simulink model "FOC_w_LTID_v2"  (R2018b)
settings: Solver=ode5  StartTime=0  StopTime=16  FixedStep=1/fs/4  MaxStep=1/fs  RelTol=1e-5  EnableMultiTasking=on
InitFcn:
  | controllers
  | model_parameters
  | KT2C = 1/(3/2)/(Npp*Lndmpm);
  | Tload = 10;
  | noise_ena = 1;
  | 
  | %SMO
  | SMO_load_gain = 15*1;  %15 corresponds to 1040
  | SMO_gain_p = 2; %1 corresponds to 70
  | smo_load_phi = 50;
  | smo_load_esf = 25; %25
  | smo_load_cutoff = 55; %75 %Hz
values from neighbouring files (symbols this model uses):
  B_m = 0.0016655    [model_parameters.m]
  C_m = 0.2295    [model_parameters.m]
  fs = 1*5e3    (= 5000)    [model_parameters.m]
  gamma = 0.001    [model_parameters.m]
  i_maxim_PM = 35    [model_parameters.m]
  J = 0.0146    [model_parameters.m]
  Ld = 2.2e-3    (= 0.0022)    [model_parameters.m]
  Lndd_ini = Lndmpm    (= 0.12258)    [model_parameters.m]
  Lndmpm = 0.12258    [model_parameters.m]
  Lq = 2.2e-3    (= 0.0022)    [model_parameters.m]
  Npp = 4    [model_parameters.m]
  Omegae_ini = 0    [model_parameters.m]
  Rs = 0.268*1    (= 0.268)    [model_parameters.m]
  Tl_const = Trat/nrat^2    (= 6.91358024691e-07)    [model_parameters.m]
  Vph = Vs*sqrt(2)    [model_parameters.m]
undefined symbols (not defined in the file or in its folder): DiscIntNeverNeededParam, Ka_speed, Ki_id, Ki_iq, Ki_speed, Kp_id, Kp_iq, Kp_speed, sigbuilder_block
libraries: simulink x2
settings Model: Creator=klu  LastModifiedBy=Barna
settings DataIOCC: LimitDataPoints=on  SaveFormat=Array  SignalLoggingSaveFormat=ModelDataLogs
settings OptimizationCC: BooleanDataType=off  ExpressionDepthLimit=2147483647  InitFltsAndDblsToZero=on  LifeSpan=inf
settings DebuggingCC: AlgebraicLoopMsg=none  SaveWithParameterizedLinksMsg=none  UnderspecifiedInitializationDetection=Classic  MergeDetectMultiDrivingBlocksExec=none  SignalResolutionControl=TryResolveAllWithWarning  MultiTaskDSMMsg=warning  MultiTaskCondExecSysMsg=none  FcnCallInpInsideContextMsg=warning  StateNameClashWarn=warning  SFUnexpectedBacktrackingDiag=warning  SFNoUnconditionalDefaultTransitionDiag=warning  SFExecutionAtInitializationDiag=none
settings HardwareCC: ProdBitPerPointer=32  ProdBitPerSizeT=32  ProdBitPerPtrDiffT=32  ProdLargestAtomicFloat=None  ProdIntDivRoundTo=Undefined  ProdEndianess=Unspecified  ProdWordSize=32  ProdHWDeviceType=32-bit Generic
settings ModelReferenceCC: PropagateSignalLabelsOutOfModel=off
settings SFSimCC: SimUseLocalCustomCode=off
settings RTWCC: RTWUseLocalCustomCode=off
settings CodeAppCC: StateflowObjectComments=on
settings GRTTargetCC: TargetFcnLib=ansi_tfl_tmw.mat  TargetLangStandard=C89/C90 (ANSI)  GeneratePreprocessorConditionals=Disable all  CombineOutputUpdateFcns=off  GRTInterface=on
settings ConfigComp: CovMetricSettings=dw  CovHtmlReporting=on  CovSaveCumulativeToWorkspaceVar=on  CovSaveSingleToWorkspaceVar=on  CovExternalEMLEnable=off  CovSFcnEnable=off

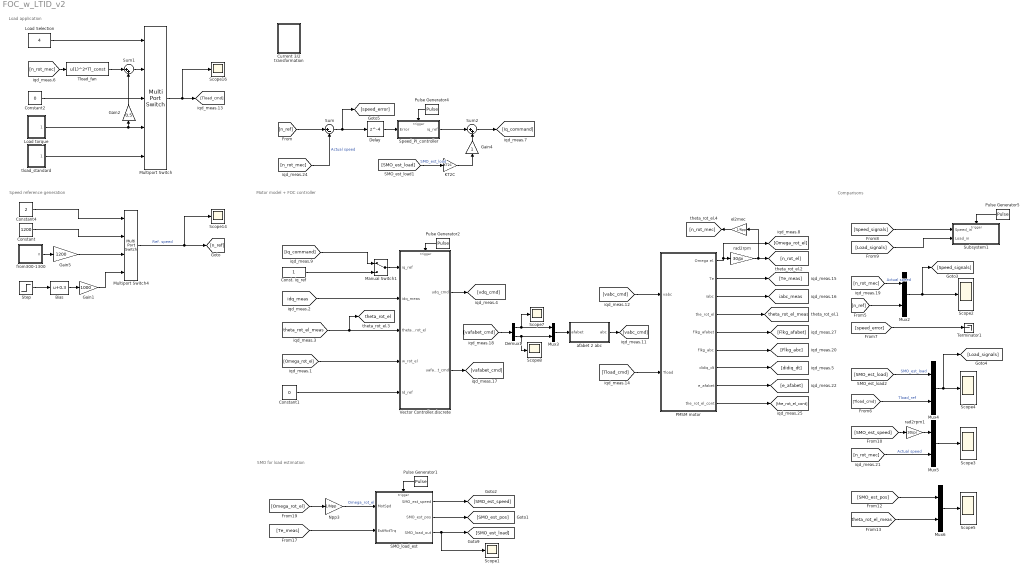
== system FOC_w_LTID_v2 ==
  note: Speed reference generation
  note: Motor model + FOC controller
  note: Load application
  note: SMO for load estimation
  note: Comparisons
  Bias : Bias  Bias=0.3
  Const. iq_ref : Constant
  Constant : Constant  Value=1200
  Constant1 : Constant  Value=0
  Constant2 : Constant  Value=0
  Constant4 : Constant  Value=2
  Current 3/2 transformation : Subsystem
      mask Display:
      | plot([0.1000    0.1357    0.1714    0.2071    0.2429    0.2786    0.3143    0.3500    0.3857    0.4214 0.4571    0.4929    0.5286    0.5643    0.6000]-0.05,0.4+0.6*[0.5000    0.5868    0.6564    0.6950    0.6950    0.6564    0.5868    0.5000    0.4132    0.3436 0.3050    0.3050    0.3436    0.4132    0.5000])
      | 
      | plot([0.1,0.9],[0.1,0.9])
      | 
      | plot([0.5,0.9],0.3*[1 1])
  Delay : Delay  DelayLength=4
  Demux1 : Demux  Outputs=2
  Gain1 : Gain  Gain=1000
  Gain2 : Gain  Gain=0.5
  Gain4 : Gain
  Gain5 : Gain  Gain=1200
  KT2C : Gain  Gain=KT2C
  Load Selection : Constant  Value=4
  Load torque : Subsystem
  Manual Switch1 : ManualSwitch
  Multiport Switch : MultiPortSwitch  Inputs=4
  Multiport Switch4 : MultiPortSwitch
  Mux{2..6} (5 alike) : Mux  Inputs=2
  Npp3 : Gain  Gain=1/Npp
  PMSM motor : Subsystem
  Pulse Generator1 : DiscretePulseGenerator  PulseType=Time based  Period=1/fs  PulseWidth=50
  Pulse Generator2 : DiscretePulseGenerator  PulseType=Time based  Period=1/fs  PulseWidth=50
  Pulse Generator4 : DiscretePulseGenerator  PulseType=Time based  Period=1/fs*2  PulseWidth=50
  Pulse Generator5 : DiscretePulseGenerator  PulseType=Time based  Period=1/fs  PulseWidth=50
  SMO_load_est : Subsystem
  Scope{1..5,7..8,14,16} (9 alike) : Scope
  Speed_PI_controller : Subsystem
  Step : Step  SampleTime=0
  Subsystem1 : Subsystem
  Sum : Sum  Inputs=|+-
  Sum1 : Sum  Inputs=|++
  Sum2 : Sum  Inputs=|++
  Terminator1 : Terminator
  Tload_fan : Fcn  Expr=u(1)^2*Tl_const
  Vector Controller.discrete : Subsystem
  afabet 2 abc : Subsystem
  el2mec : Gain  Gain=1/Npp
  "from300-1300 " : Subsystem  Tag=STV Subsys  LoadFcn=sigbuilder_block('load');  StartFcn=sigbuilder_block('start');  StopFcn=sigbuilder_block('stop');  ClipboardFcn=sigbuilder_block('clipboard');  mask(Sigbuilder block){tuvar=[0:10]}
      mask help: Sigbuilder GUI
      mask init:
      | if ~strcmp(get_param(bdroot(gcbh),'SimulationStatus'),'stopped') tuvar = sigbuilder_block('maskInit'); end
      settings: CopyFcn=sigbuilder_block('copy');  DeleteFcn=sigbuilder_block('delete');  ModelCloseFcn=sigbuilder_block('modelClose');  PreSaveFcn=sigbuilder_block('preSave');  PauseFcn=sigbuilder_block('pause')  ContinueFcn=sigbuilder_block('continue')  NameChangeFcn=sigbuilder_block('namechange');  OpenFcn=sigbuilder_block('open',[0 0 1096.2 591.6 ]);  CloseFcn=sigbuilder_block('close');
      mask Display: plot(0, 0, 100, 100,[2, 2, 32, 32, 2], [68, 8, 8, 68, 68],[32, 2], [38, 38], [32, 19, 2],[53, 60, 44], [32, 17, 17, 2],[16, 16, 31, 31]);txt = getActiveGroup(gcbh);text(2, 100, txt,'verticalAlignment', 'top');
  rad2rpm : Gain  Gain=30/pi
  rad2rpm1 : Gain  Gain=30/pi
  tload_standard : Subsystem
  tag scope: iabc_meas=global, theta_rot_el=global, theta_rot_el_meas=global
  wires:
  Manual Switch1/1 -> Vector Controller.discrete/1(iq_ref)
  Const. iq_ref/1 -> Manual Switch1/2
  [idq_meas] -> Vector Controller.discrete/2(idq_meas)
  Vector Controller.discrete/1(udq_cmd) -> [vdq_cmd]
  Vector Controller.discrete/2(uafabet_cmd) -> [vafabet_cmd]
  Constant2/1 -> Multiport Switch/3
  Load torque/1(T_load) -> Multiport Switch/4, Gain2/1
  Multiport Switch/1 -> Scope16/1, [Tload_cmd]
  [n_rot_mec] -> Tload_fan/1
  Load Selection/1 -> Multiport Switch/1
  Pulse Generator2/1 -> Vector Controller.discrete/Trigger
  Sum1/1 -> Multiport Switch/2
  Tload_fan/1 -> Sum1/1
  Constant1/1 -> Vector Controller.discrete/5(Id_ref)
  Gain2/1 -> Sum1/2
  PMSM motor/2(Te) -> [Te_meas]
  PMSM motor/1(Omega el.) -> [Omega_rot_el], rad2rpm/1
  [vabc_cmd] -> PMSM motor/1(vabc)
  rad2rpm/1 -> el2mec/1, [n_rot_el]
  PMSM motor/4(the_rot_el) -> [theta_rot_el_meas]
  PMSM motor/5(Flkg_afabet) -> [Flkg_afabet]
  PMSM motor/6(Flkg_abc) -> [Flkg_abc]
  [Tload_cmd] -> PMSM motor/2(Tload)
  PMSM motor/3(iabc) -> [iabc_meas]
  PMSM motor/7(didiq_dt) -> [didiq_dt]
  Demux1/2 -> Mux3/2, Scope8/1
  Demux1/1 -> Scope7/1, Mux3/1
  [vafabet_cmd] -> Demux1/1
  afabet 2 abc/1(abc) -> [vabc_cmd]
  Mux3/1 -> afabet 2 abc/1(afabet)
  el2mec/1 -> [n_rot_mec]
  [Iq_command] -> Manual Switch1/1
  [theta_rot_el_meas] -> [theta_rot_el], Vector Controller.discrete/3(theta_rot_el)
  [Omega_rot_el] -> Vector Controller.discrete/4(w_rot_el)
  PMSM motor/8(e_afabet) -> [e_afabet]
  Multiport Switch4/1 -> Scope14/1, [n_ref]  "Ref. speed"
  Pulse Generator4/1 -> Speed_PI_controller/Trigger
  Sum/1 -> Delay/1, [speed_error]
  Constant4/1 -> Multiport Switch4/1
  Constant/1 -> Multiport Switch4/2
  PMSM motor/9(the_rot_el_cont) -> [the_rot_el_cont]
  Delay/1 -> Speed_PI_controller/1(Error)
  tload_standard/1(T_load) -> Multiport Switch/5
  "from300-1300 "/1(n) -> Gain5/1
  [n_rot_mec] -> Sum/2  "Actual speed"
  [n_ref] -> Sum/1
  Gain5/1 -> Multiport Switch4/3
  Step/1 -> Bias/1
  Bias/1 -> Gain1/1
  Gain1/1 -> Multiport Switch4/4
  [Omega_rot_el] -> Npp3/1
  [Te_meas] -> SMO_load_est/2(EstMotTrq)
  Npp3/1 -> SMO_load_est/1(MotSpd)  "Omega_rot_el"
  Pulse Generator1/1 -> SMO_load_est/Trigger
  Speed_PI_controller/1(iq_ref) -> Sum2/1
  Sum2/1 -> [Iq_command]
  Gain4/1 -> Sum2/2
  [SMO_est_load] -> KT2C/1  "SMO_est_load"
  KT2C/1 -> Gain4/1
  [speed_error] -> Terminator1/1
  Mux4/1 -> Scope4/1, [Load_signals]
  [SMO_est_load] -> Mux4/1  "SMO_est_load"
  [Tload_cmd] -> Mux4/2  "Tload_ref"
  Mux2/1 -> [Speed_signals], Scope2/1
  [Speed_signals] -> Subsystem1/1(Speed_in)
  [Load_signals] -> Subsystem1/2(Load_in)
  Pulse Generator5/1 -> Subsystem1/Trigger
  [theta_rot_el_meas] -> Mux6/2
  [n_ref] -> Mux2/2
  [SMO_est_pos] -> Mux6/1
  [n_rot_mec] -> Mux2/1  "Actual speed"
  Mux5/1 -> Scope3/1
  [n_rot_mec] -> Mux5/2  "Actual speed"
  [SMO_est_speed] -> rad2rpm1/1
  rad2rpm1/1 -> Mux5/1
  Mux6/1 -> Scope5/1
  SMO_load_est/2(SMO_est_pos) -> [SMO_est_pos]
  SMO_load_est/1(SMO_est_speed) -> [SMO_est_speed]
  SMO_load_est/3(SMO_load_out) -> Scope1/1, [SMO_est_load]

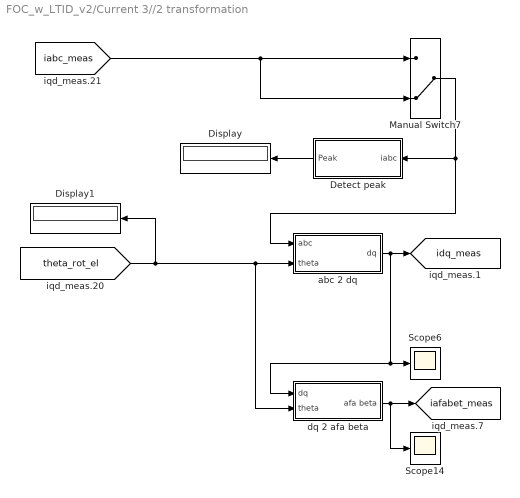
== system FOC_w_LTID_v2/Current 3//2 transformation ==
  Detect peak : Subsystem
  Display : Display
  Display1 : Display
  Manual Switch7 : ManualSwitch  CurrentSetting=0
  Scope14 : Scope
  Scope6 : Scope
  abc 2 dq : Subsystem
  dq 2 afa beta : Subsystem
  tag scope: iafabet_meas=global, idq_meas=global
  wires:
  abc 2 dq/1(dq) -> [idq_meas], Scope6/1, dq 2 afa beta/1(dq)
  dq 2 afa beta/1(afa beta) -> [iafabet_meas], Scope14/1
  Manual Switch7/1 -> abc 2 dq/1(abc), Detect peak/1(iabc)
  Detect peak/1(Peak) -> Display/1
  [theta_rot_el] -> abc 2 dq/2(theta), dq 2 afa beta/2(theta), Display1/1
  [iabc_meas] -> Manual Switch7/1, Manual Switch7/2

== system FOC_w_LTID_v2/Load torque ==
  Add : Sum  Inputs=+++
  Step Load torque 1 : Step  Time=1.5  After=Tload  SampleTime=0
  Step Load torque2 : Step  Time=2  After=-Tload  SampleTime=0
  Tload : Constant  Value=0
  T_load : Outport
  wires:
  Tload/1 -> Add/1
  Step Load torque 1/1 -> Add/2
  Step Load torque2/1 -> Add/3
  Add/1 -> T_load/1

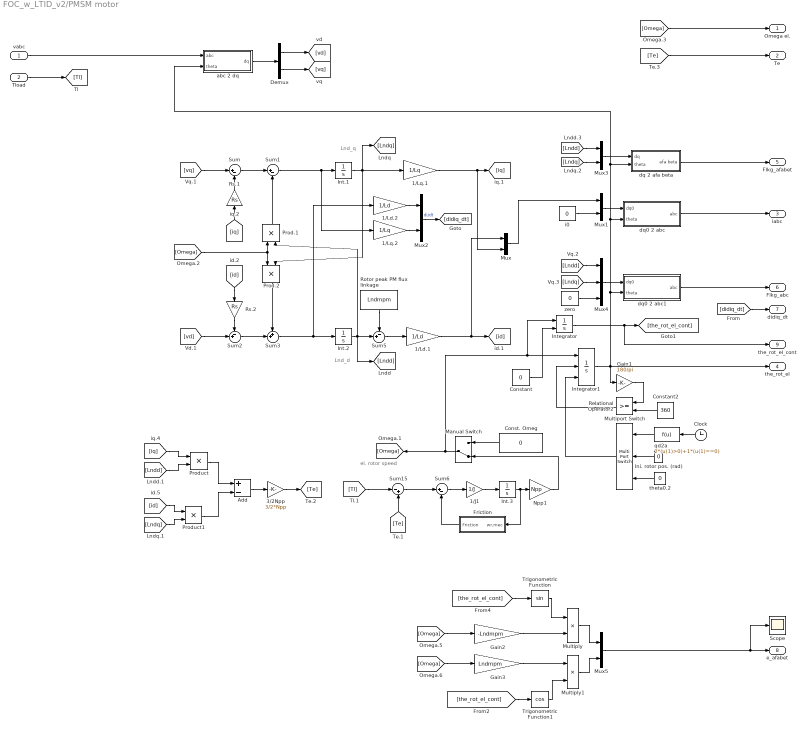
== system FOC_w_LTID_v2/PMSM motor ==
  note: Lnd_d
  note: Lnd_q
  note: el. rotor speed
  vabc : Inport
  Tload : Inport  Port=2
  1/J1 : Gain  Gain=1/J
  1/Ld.1 : Gain  Gain=1/Ld
  1/Ld.2 : Gain  Gain=1/Ld
  1/Lq.1 : Gain  Gain=1/Lq
  1/Lq.2 : Gain  Gain=1/Lq
  3/2Npp : Gain  Gain=3/2*Npp
  Add : Sum  Inputs=+-
  Clock : Clock
  Const. Omeg : Constant  Value=0
  Constant : Constant  Value=0
  Constant2 : Constant  Value=360
  Demux : Demux  Outputs=2
  Friction : Subsystem
  Gain1 : Gain  Gain=180/pi
  Gain2 : Gain  Gain=-Lndmpm
  Gain3 : Gain  Gain=Lndmpm
  Ini. rotor pos. (rad) : Constant  Value=0
  Int.1 : Integrator
  Int.2 : Integrator  InitialCondition=Lndd_ini
  Int.3 : Integrator  InitialCondition=Omegae_ini/Npp
  Integrator : Integrator  InitialConditionSource=external
  Integrator1 : Integrator  ExternalReset=rising  InitialConditionSource=external  InitialCondition=pi/3
  Manual Switch : ManualSwitch  CurrentSetting=0
  Multiply : Product
  Multiply1 : Product
  Multiport Switch : MultiPortSwitch  Inputs=2
  Mux{,1..3,5} (5 alike) : Mux  Inputs=2
  Mux4 : Mux  Inputs=3
  Npp1 : Gain  Gain=Npp
  Prod.1 : Product  RndMeth=Zero
  Prod.2 : Product  RndMeth=Zero
  Product : Product  RndMeth=Zero
  Product1 : Product  RndMeth=Zero
  Relational Operator2 : RelationalOperator  OutDataTypeStr=boolean  RndMeth=Nearest
  Rotor peak PM flux linkage : Constant  Value=Lndmpm
  Rs.1 : Gain  Gain=Rs
  Rs.2 : Gain  Gain=Rs
  Scope : Scope
  Sum : Sum  Inputs=|+-
  Sum1 : Sum  Inputs=|+-
  Sum15 : Sum  Inputs=|-+
  Sum2 : Sum  Inputs=-+|
  Sum3 : Sum  Inputs=++|
  Sum5 : Sum  Inputs=-+|
  Sum6 : Sum  Inputs=|+-
  Trigonometric Function : Trigonometry
  Trigonometric Function1 : Trigonometry  Operator=cos
  abc 2 dq : Subsystem
  dq 2 afa beta : Subsystem
  dq0 2 abc : Subsystem
  dq0 2 abc1 : Subsystem
  i0 : Constant  Value=0
  qd2a : Fcn  Expr=2*(u(1)>0)+1*(u(1)==0)
  theta0.2 : Constant  Value=0
  zero : Constant  Value=0
  Omega el. : Outport
  Te : Outport  Port=2
  iabc : Outport  Port=3
  the_rot_el : Outport  Port=4
  Flkg_afabet : Outport  Port=5
  Flkg_abc : Outport  Port=6
  didiq_dt : Outport  Port=7
  e_afabet : Outport  Port=8
  the_rot_el_cont : Outport  Port=9
  wires:
  3/2Npp/1 -> [Te]
  Add/1 -> 3/2Npp/1
  Sum5/1 -> 1/Ld.1/1
  Rotor peak PM flux linkage/1 -> Sum5/1
  [Omega] -> Omega el./1
  [Te] -> Te/1
  Product1/1 -> Add/2
  Product/1 -> Add/1
  [Lndq] -> Product1/2
  [id] -> Product1/1
  [Te] -> Sum15/2
  [Tl] -> Sum15/1
  Mux/1 -> Mux1/1
  [Omega] -> Prod.2/1, Prod.1/1
  Sum3/1 -> Int.2/1, 1/Ld.2/1
  Prod.2/1 -> Sum3/1
  Sum2/1 -> Sum3/2
  [id] -> Rs.2/1
  Rs.2/1 -> Sum2/1
  [vd] -> Sum2/2
  1/Ld.1/1 -> [id], Mux/1
  Int.2/1 -> [Lndd], Sum5/2, Prod.1/2
  [iq] -> Rs.1/1
  1/Lq.1/1 -> [iq], Mux/2
  Prod.1/1 -> Sum1/2
  Sum1/1 -> Int.1/1, 1/Lq.2/1
  Int.1/1 -> 1/Lq.1/1, Prod.2/2, [Lndq]
  Sum/1 -> Sum1/1
  Rs.1/1 -> Sum/2
  [vq] -> Sum/1
  Tload/1 -> [Tl]
  Demux/2 -> [vq]
  Demux/1 -> [vd]
  i0/1 -> Mux1/2
  Mux1/1 -> dq0 2 abc/1(dq0)
  dq0 2 abc/1(abc) -> iabc/1
  vabc/1 -> abc 2 dq/1(abc)
  abc 2 dq/1(dq) -> Demux/1
  Integrator1/1 -> the_rot_el/1, dq0 2 abc/2(theta), dq 2 afa beta/2(theta), abc 2 dq/2(theta), dq0 2 abc1/2(theta), Gain1/1
  1/Ld.2/1 -> Mux2/1
  1/Lq.2/1 -> Mux2/2
  Mux3/1 -> dq 2 afa beta/1(dq)
  [Lndd] -> Mux3/1
  [Lndq] -> Mux3/2
  dq 2 afa beta/1(afa beta) -> Flkg_afabet/1
  [Lndd] -> Mux4/1
  [Lndq] -> Mux4/2
  Mux4/1 -> dq0 2 abc1/1(dq0)
  dq0 2 abc1/1(abc) -> Flkg_abc/1
  zero/1 -> Mux4/3
  Gain1/1 -> Relational Operator2/1
  Constant2/1 -> Relational Operator2/2
  [iq] -> Product/1
  [Lndd] -> Product/2
  Relational Operator2/1 -> Integrator1/2
  Ini. rotor pos. (rad)/1 -> Multiport Switch/2
  theta0.2/1 -> Multiport Switch/3
  qd2a/1 -> Multiport Switch/1
  Clock/1 -> qd2a/1
  Multiport Switch/1 -> Integrator1/3
  Const. Omeg/1 -> Manual Switch/1
  Npp1/1 -> Manual Switch/2
  Manual Switch/1 -> Integrator/1, Integrator1/1, [Omega]
  Friction/1(Friction) -> Sum6/2
  Int.3/1 -> Friction/1(wr,mec), Npp1/1
  Sum6/1 -> 1/J1/1
  1/J1/1 -> Int.3/1
  Sum15/1 -> Sum6/1
  Mux5/1 -> Scope/1, e_afabet/1
  Trigonometric Function1/1 -> Multiply1/2
  [Omega] -> Gain2/1
  [the_rot_el_cont] -> Trigonometric Function1/1
  Gain3/1 -> Multiply1/1
  Multiply1/1 -> Mux5/2
  [the_rot_el_cont] -> Trigonometric Function/1
  Multiply/1 -> Mux5/1
  [Omega] -> Gain3/1
  Gain2/1 -> Multiply/2
  Trigonometric Function/1 -> Multiply/1
  Integrator/1 -> the_rot_el_cont/1, [the_rot_el_cont]
  Constant/1 -> Integrator/2
  Mux2/1 -> [didiq_dt]  "di/dt"
  [didiq_dt] -> didiq_dt/1

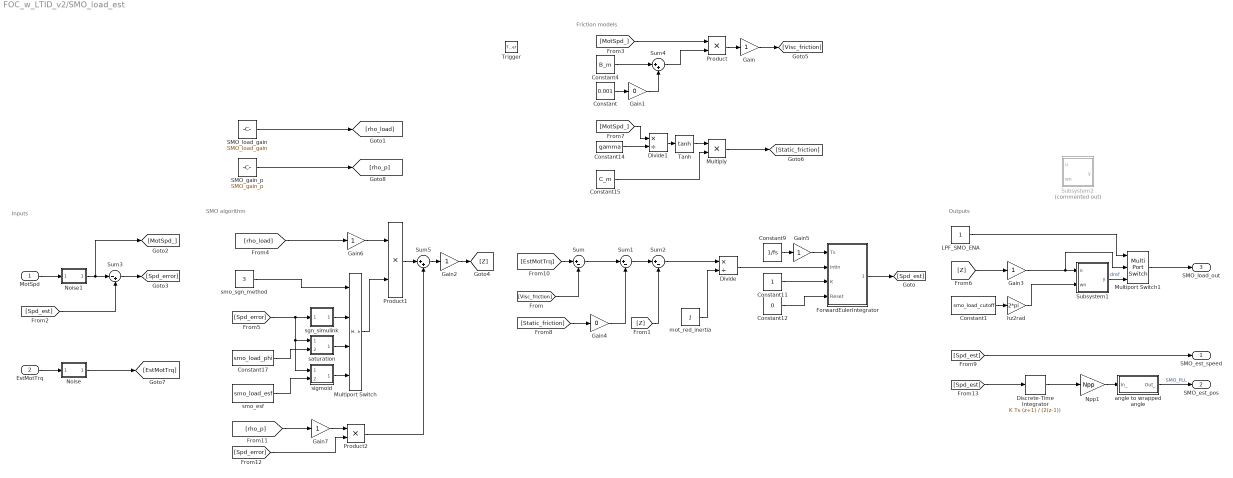
== system FOC_w_LTID_v2/SMO_load_est ==
  note: Inputs
  note: Outputs
  note: Friction models
  note: SMO algorithm
  MotSpd : Inport
  EstMotTrq : Inport  Port=2
  Trigger : TriggerPort  VariantControl=(inherit)
  Constant : Constant  Value=0.001
  Constant1 : Constant  Value=smo_load_cutoff
  Constant11 : Constant
  Constant12 : Constant  Value=0
  Constant14 : Constant  Value=gamma
  Constant15 : Constant  Value=C_m
  Constant17 : Constant  Value=smo_load_phi
  Constant4 : Constant  Value=B_m
  Constant9 : Constant  Value=1/fs
  Discrete-Time Integrator : DiscreteIntegrator  IntegratorMethod=Integration: Trapezoidal  SampleTime=-1  ICPrevOutput=DiscIntNeverNeededParam  ICPrevScaledInput=DiscIntNeverNeededParam
  Divide : Product  Inputs=*/
  Divide1 : Product  Inputs=*/
  ForwardEulerIntegrator : Subsystem
  Gain{,2..3,5..7} (6 alike) : Gain
  Gain1 : Gain  Gain=0
  Gain4 : Gain  Gain=0
  LPF_SMO_ENA : Constant
  Multiply : Product
  Multiport Switch : MultiPortSwitch
  Multiport Switch1 : MultiPortSwitch  DataPortOrder=Zero-based contiguous  Inputs=2  zeroidx=on
  Noise : Subsystem
  Noise1 : Subsystem
  Npp1 : Gain  Gain=Npp
  Product : Product
  Product1 : Product
  Product2 : Product
  SMO_gain_p : Constant  Value=SMO_gain_p
  SMO_load_gain : Constant  Value=SMO_load_gain
  Subsystem1 : Subsystem
  Subsystem2 : Subsystem  Commented=on
  Sum : Sum  Inputs=|+-
  Sum1 : Sum  Inputs=|+-
  Sum2 : Sum  Inputs=|+-
  Sum3 : Sum  Inputs=|-+
  Sum4 : Sum  Inputs=|++
  Sum5 : Sum  Inputs=|++
  Tanh : Trigonometry  Operator=tanh
  angle to wrapped angle : Subsystem
  hz2rad : Gain  Gain=2*pi
  mot_red_inertia : Constant  Value=J
  saturation : Subsystem
  sgn_simulink : Subsystem
  sigmoid : Subsystem
  smo_esf : Constant  Value=smo_load_esf
  smo_sgn_method : Constant  Value=3
  SMO_est_speed : Outport
  SMO_est_pos : Outport  Port=2
  SMO_load_out : Outport  Port=3
  wires:
  [Visc_friction] -> Sum/2
  Sum/1 -> Sum1/1
  mot_red_inertia/1 -> Divide/2
  [Spd_est] -> Sum3/2
  MotSpd/1 -> Noise1/1(In1)
  Sum3/1 -> [Spd_error]
  Product/1 -> Gain/1
  [MotSpd_] -> Product/1
  Gain/1 -> [Visc_friction]
  Constant4/1 -> Sum4/1
  Constant/1 -> Gain1/1
  Gain1/1 -> Sum4/2
  Sum4/1 -> Product/2
  Gain2/1 -> [Z]
  [rho_load] -> Gain6/1
  smo_sgn_method/1 -> Multiport Switch/1
  sgn_simulink/1(Out_) -> Multiport Switch/2
  saturation/1(Out_) -> Multiport Switch/3
  sigmoid/1(Out_) -> Multiport Switch/4
  Multiport Switch/1 -> Product1/2
  Constant17/1 -> saturation/2(phi)
  smo_esf/1 -> sigmoid/2(esf)
  [Spd_error] -> sgn_simulink/1(Sigma), sigmoid/1(Sigma), saturation/1(Sigma)
  Constant1/1 -> hz2rad/1
  Gain3/1 -> Multiport Switch1/2, Subsystem1/1(u)
  hz2rad/1 -> Subsystem1/2(wn)
  Constant14/1 -> Divide1/2
  Constant15/1 -> Multiply/2
  Divide1/1 -> Tanh/1
  Tanh/1 -> Multiply/1
  [MotSpd_] -> Divide1/1
  Multiply/1 -> [Static_friction]
  [Static_friction] -> Gain4/1
  Gain4/1 -> Sum1/2
  Constant12/1 -> ForwardEulerIntegrator/4(Reset)
  Constant11/1 -> ForwardEulerIntegrator/3(K)
  Constant9/1 -> Gain5/1
  Gain5/1 -> ForwardEulerIntegrator/1(Ts)
  ForwardEulerIntegrator/1(IntOut_) -> [Spd_est]
  Subsystem1/1(y) -> Multiport Switch1/3  "dref"
  Multiport Switch1/1 -> SMO_load_out/1
  LPF_SMO_ENA/1 -> Multiport Switch1/1
  [Spd_est] -> SMO_est_speed/1
  EstMotTrq/1 -> Noise/1(In1)
  [EstMotTrq] -> Sum/1
  SMO_load_gain/1 -> [rho_load]
  Noise/1(Out1) -> [EstMotTrq]
  Noise1/1(Out1) -> [MotSpd_], Sum3/1
  Sum1/1 -> Sum2/1
  Sum2/1 -> Divide/1
  Divide/1 -> ForwardEulerIntegrator/2(IntIn)
  [Z] -> Sum2/2
  [Z] -> Gain3/1
  Product1/1 -> Sum5/1
  Sum5/1 -> Gain2/1
  [rho_p] -> Gain7/1
  [Spd_error] -> Product2/2
  Product2/1 -> Sum5/2
  SMO_gain_p/1 -> [rho_p]
  Npp1/1 -> angle to wrapped angle/1(In_)
  Discrete-Time Integrator/1 -> Npp1/1
  [Spd_est] -> Discrete-Time Integrator/1
  angle to wrapped angle/1(Out_) -> SMO_est_pos/1  "SMO_PLL"
  Gain6/1 -> Product1/1
  Gain7/1 -> Product2/1

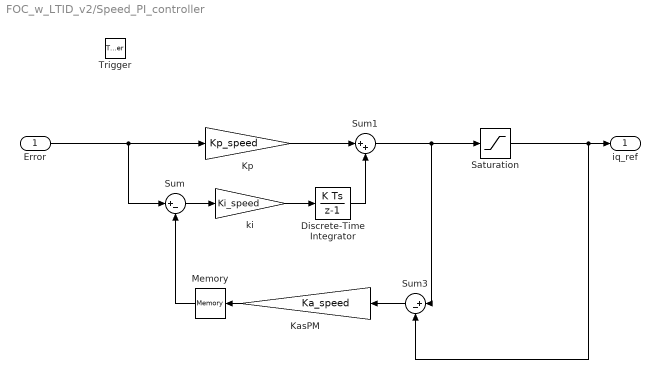
== system FOC_w_LTID_v2/Speed_PI_controller ==
  Error : Inport
  Trigger : TriggerPort  VariantControl=(inherit)
  Discrete-Time Integrator : DiscreteIntegrator  SampleTime=-1  ICPrevOutput=DiscIntNeverNeededParam  ICPrevScaledInput=DiscIntNeverNeededParam
  KasPM : Gain  Gain=Ka_speed
  Kp : Gain  Gain=Kp_speed
  Memory : Memory  InheritSampleTime=on
  Saturation : Saturate  UpperLimit=i_maxim_PM  LowerLimit=-i_maxim_PM
  Sum : Sum  Inputs=|+-
  Sum1 : Sum  Inputs=|++
  Sum3 : Sum  Inputs=|+-
  ki : Gain  Gain=Ki_speed
  iq_ref : Outport
  wires:
  Kp/1 -> Sum1/1
  ki/1 -> Discrete-Time Integrator/1
  Discrete-Time Integrator/1 -> Sum1/2
  Error/1 -> Sum/1, Kp/1
  KasPM/1 -> Memory/1
  Memory/1 -> Sum/2
  Sum1/1 -> Sum3/1, Saturation/1
  Sum3/1 -> KasPM/1
  Saturation/1 -> iq_ref/1, Sum3/2
  Sum/1 -> ki/1

== system FOC_w_LTID_v2/Subsystem1 ==
  Speed_in : Inport
  Load_in : Inport  Port=2
  Trigger : TriggerPort  VariantControl=Variant  PortDimensions=1
  To Workspace : ToWorkspace  VariableName=Speed_in  SaveFormat=Structure With Time  SampleTime=-1
  To Workspace1 : ToWorkspace  VariableName=SMO_EstLoad  SaveFormat=Structure With Time  SampleTime=-1
  wires:
  Speed_in/1 -> To Workspace/1
  Load_in/1 -> To Workspace1/1

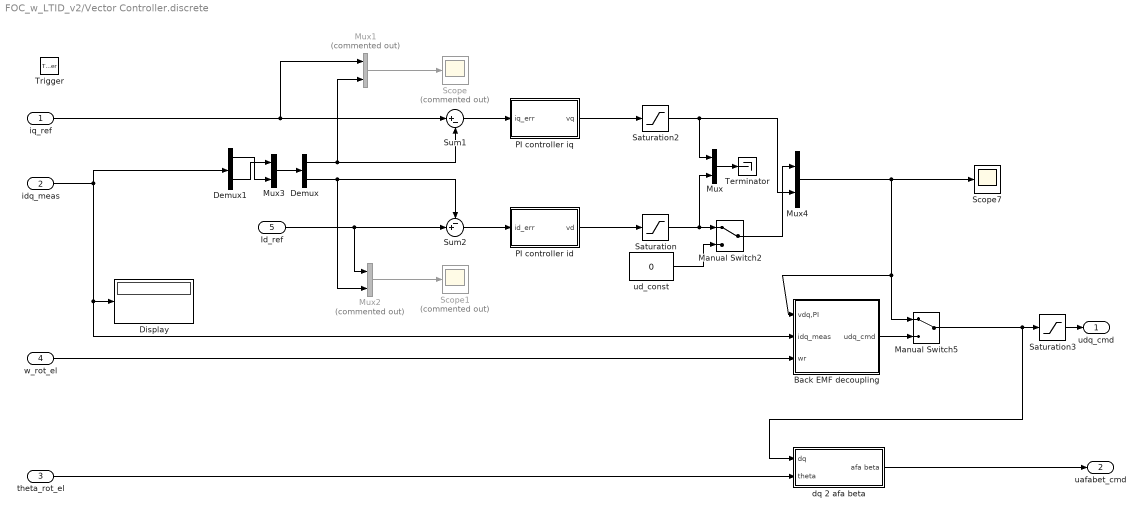
== system FOC_w_LTID_v2/Vector Controller.discrete ==
  iq_ref : Inport
  idq_meas : Inport  Port=2
  theta_rot_el : Inport  Port=3
  w_rot_el : Inport  Port=4
  Id_ref : Inport  Port=5
  Trigger : TriggerPort  VariantControl=(inherit)
  Back EMF decoupling : Subsystem
  Demux : Demux  Outputs=2
  Demux1 : Demux  Outputs=2
  Display : Display
  Manual Switch2 : ManualSwitch
  Manual Switch5 : ManualSwitch
  Mux : Mux  Inputs=2
  Mux1 : Mux  Commented=on  Inputs=2
  Mux2 : Mux  Commented=on  Inputs=2
  Mux3 : Mux  Inputs=2
  Mux4 : Mux  Inputs=2
  PI controller id : Subsystem
  PI controller iq : Subsystem
  Saturation : Saturate  UpperLimit=Vph  LowerLimit=-Vph
  Saturation2 : Saturate  UpperLimit=Vph  LowerLimit=-Vph
  Saturation3 : Saturate  UpperLimit=Vph  LowerLimit=-Vph
  Scope : Scope  Commented=on
  Scope1 : Scope  Commented=on
  Scope7 : Scope
  Sum1 : Sum  Inputs=|+-
  Sum2 : Sum  Inputs=-+|
  Terminator : Terminator
  dq 2 afa beta : Subsystem
  ud_const : Constant  Value=0
  udq_cmd : Outport
  uafabet_cmd : Outport  Port=2
  wires:
  Id_ref/1 -> Sum2/2, Mux2/1
  Saturation/1 -> Mux/2, Manual Switch2/1
  Mux/1 -> Terminator/1
  PI controller iq/1(vq) -> Saturation2/1
  Demux/1 -> Sum1/2, Mux1/2
  PI controller id/1(vd) -> Saturation/1
  Demux/2 -> Sum2/1, Mux2/2
  Sum1/1 -> PI controller iq/1(iq_err)
  Sum2/1 -> PI controller id/1(id_err)
  iq_ref/1 -> Sum1/1, Mux1/1
  Saturation2/1 -> Mux/1, Mux4/2
  Manual Switch2/1 -> Mux4/1
  ud_const/1 -> Manual Switch2/2
  Demux1/2 -> Mux3/1
  Demux1/1 -> Mux3/2
  theta_rot_el/1 -> dq 2 afa beta/2(theta)
  w_rot_el/1 -> Back EMF decoupling/3(wr)
  Back EMF decoupling/1(udq_cmd) -> Manual Switch5/2
  Mux4/1 -> Scope7/1, Manual Switch5/1, Back EMF decoupling/1(vdq,PI)
  Manual Switch5/1 -> dq 2 afa beta/1(dq), Saturation3/1
  Mux3/1 -> Demux/1
  idq_meas/1 -> Demux1/1, Display/1, Back EMF decoupling/2(idq_meas)
  Saturation3/1 -> udq_cmd/1
  dq 2 afa beta/1(afa beta) -> uafabet_cmd/1
  Mux1/1 -> Scope/1
  Mux2/1 -> Scope1/1

== system FOC_w_LTID_v2/afabet 2 abc ==
  afabet : Inport
  Constant : Constant  Value=0
  Mux1 : Mux  Inputs=2
  Mux2 : Mux  Inputs=3
  qd2a : Fcn  Expr=u(1)+u(3)
  qd2b : Fcn  Expr=u(1)*cos(2/3*pi)+u(2)*sin(2/3*pi)+u(3)
  qd2c : Fcn  Expr=u(1)*cos(2/3*pi)-u(2)*sin(2/3*pi)+u(3)
  abc : Outport
  wires:
  Constant/1 -> Mux1/2
  qd2c/1 -> Mux2/3
  afabet/1 -> Mux1/1
  Mux1/1 -> qd2c/1, qd2b/1, qd2a/1
  qd2a/1 -> Mux2/1
  qd2b/1 -> Mux2/2
  Mux2/1 -> abc/1

== system FOC_w_LTID_v2/from300-1300  ==
  Demux : Demux  Tag=STV Demux  Outputs=1
  FromWs : FromWorkspace  Tag=STV FromWs  VariableName=tuvar  SampleTime=0
      SigBuilderData=|
      | common.afterFinalStr = 'Extrapolate'
      | common.sampleTime = 0
      | dataSet.timeRange = [0 16]
      | dataSet.name = 'Group 1'
      | sbobj.Groups.Name = 'Group 1'
      | sbobj.Groups.Signals.Name = 'n'
      | sbobj.Groups.Signals.XData = [0 1 1.5 5 5.5 11 11.5 15 15.5 16]
      | sbobj.Groups.Signals.YData = [0.3 0.3 1.3 1.3 0.3 0.3 1.3 1.3 0.3 0.3]
      | sbobj.Groups.TimeRange = [0 16]
  n : Outport  Tag=STV Outport
  wires:
  Demux/1 -> n/1
  FromWs/1 -> Demux/1

== system FOC_w_LTID_v2/tload_standard ==
  Add : Sum  Inputs=+++++
  Step Load torque 1 : Step  Time=3  After=Tload  SampleTime=0
  Step Load torque1 : Step  Time=9  After=Tload  SampleTime=0
  Step Load torque2 : Step  Time=7  After=-Tload  SampleTime=0
  Step Load torque3 : Step  Time=13  After=-Tload  SampleTime=0
  Tload_ini : Constant  Value=0
  T_load : Outport
  wires:
  Tload_ini/1 -> Add/1
  Step Load torque 1/1 -> Add/2
  Step Load torque2/1 -> Add/3
  Add/1 -> T_load/1
  Step Load torque1/1 -> Add/4
  Step Load torque3/1 -> Add/5

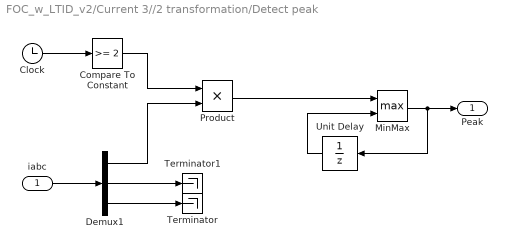
== system FOC_w_LTID_v2/Current 3//2 transformation/Detect peak ==
  iabc : Inport
  Clock : Clock
  Compare To Constant : simulink/Logic and Bit Operations/Compare To Constant  relop=>=  const=2  OutDataTypeStr=uint8  ZeroCross=off
  Demux1 : Demux  Outputs=3
  MinMax : MinMax  Function=max  Inputs=2
  Product : Product  RndMeth=Zero
  Terminator : Terminator
  Terminator1 : Terminator
  Unit Delay : UnitDelay  SampleTime=-1
  Peak : Outport
  wires:
  iabc/1 -> Demux1/1
  Demux1/3 -> Terminator/1
  Demux1/2 -> Terminator1/1
  Clock/1 -> Compare To Constant/1
  Compare To Constant/1 -> Product/1
  Demux1/1 -> Product/2
  MinMax/1 -> Peak/1, Unit Delay/1
  Product/1 -> MinMax/1
  Unit Delay/1 -> MinMax/2

== system FOC_w_LTID_v2/Current 3//2 transformation/abc 2 dq ==
  abc : Inport
  theta : Inport  Port=2
  Mux1 : Mux  Inputs=2
  Mux2 : Mux  Inputs=2
  abc2d : Fcn  Expr=2/3*(u(1)*cos(u(4))+u(2)*cos(u(4)-2*pi/3)+u(3)*cos(u(4)-4*pi/3))
  abc2q : Fcn  Expr=-1*2/3*(u(1)*sin(u(4))+u(2)*sin(u(4)-2*pi/3)+u(3)*sin(u(4)-4*pi/3))
  dq : Outport
  wires:
  Mux2/1 -> dq/1
  abc2q/1 -> Mux2/2
  abc2d/1 -> Mux2/1
  Mux1/1 -> abc2q/1, abc2d/1
  theta/1 -> Mux1/2
  abc/1 -> Mux1/1

== system FOC_w_LTID_v2/Current 3//2 transformation/dq 2 afa beta ==
  dq : Inport
  theta : Inport  Port=2
  Mux1 : Mux  Inputs=2
  Mux2 : Mux  Inputs=2
  dq2afa : Fcn  Expr=u(1)*cos(u(3))-u(2)*sin(u(3))
  dq2beta : Fcn  Expr=u(1)*sin(u(3))+u(2)*cos(u(3))
  afa beta : Outport
  wires:
  dq/1 -> Mux1/1
  theta/1 -> Mux1/2
  Mux1/1 -> dq2beta/1, dq2afa/1
  dq2afa/1 -> Mux2/1
  dq2beta/1 -> Mux2/2
  Mux2/1 -> afa beta/1

== system FOC_w_LTID_v2/PMSM motor/Friction ==
  wr,mec : Inport
  Constant14 : Constant  Value=gamma
  Constant15 : Constant  Value=C_m
  Divide : Product  Inputs=*/
  Gain : Gain  Gain=0
  Gain2 : Gain  Gain=B_m
  Multiply : Product
  Sum : Sum  Inputs=|++
  Tanh : Trigonometry  Operator=tanh
  Friction : Outport
  wires:
  Divide/1 -> Tanh/1
  Tanh/1 -> Multiply/1
  Constant15/1 -> Multiply/2
  Constant14/1 -> Divide/2
  wr,mec/1 -> Divide/1, Gain2/1
  Multiply/1 -> Gain/1
  Gain2/1 -> Sum/1
  Sum/1 -> Friction/1
  Gain/1 -> Sum/2

== system FOC_w_LTID_v2/PMSM motor/abc 2 dq ==
  abc : Inport
  theta : Inport  Port=2
  Mux1 : Mux  Inputs=2
  Mux2 : Mux  Inputs=2
  abc2d : Fcn  Expr=-1*2/3*(u(1)*sin(u(4))+u(2)*sin(u(4)-2*pi/3)+u(3)*sin(u(4)-4*pi/3))
  abc2q : Fcn  Expr=2/3*(u(1)*cos(u(4))+u(2)*cos(u(4)-2*pi/3)+u(3)*cos(u(4)-4*pi/3))
  dq : Outport
  wires:
  Mux2/1 -> dq/1
  abc2d/1 -> Mux2/2
  abc2q/1 -> Mux2/1
  Mux1/1 -> abc2d/1, abc2q/1
  theta/1 -> Mux1/2
  abc/1 -> Mux1/1

== system FOC_w_LTID_v2/PMSM motor/dq 2 afa beta ==
  dq : Inport
  theta : Inport  Port=2
  Mux1 : Mux  Inputs=2
  Mux2 : Mux  Inputs=2
  dq2afa : Fcn  Expr=u(1)*cos(u(3))-u(2)*sin(u(3))
  dq2beta : Fcn  Expr=u(1)*sin(u(3))+u(2)*cos(u(3))
  afa beta : Outport
  wires:
  dq/1 -> Mux1/1
  theta/1 -> Mux1/2
  Mux1/1 -> dq2beta/1, dq2afa/1
  dq2afa/1 -> Mux2/1
  dq2beta/1 -> Mux2/2
  Mux2/1 -> afa beta/1

== system FOC_w_LTID_v2/PMSM motor/dq0 2 abc ==
  dq0 : Inport
  theta : Inport  Port=2
  Mux1 : Mux  Inputs=2
  Mux2 : Mux  Inputs=3
  qd2a : Fcn  Expr=u(1)*cos(u(4))-u(2)*sin(u(4))+u(3)
  qd2b : Fcn  Expr=u(1)*cos(u(4)-2/3*pi)-u(2)*sin(u(4)-2/3*pi)+u(3)
  qd2c : Fcn  Expr=u(1)*cos(u(4)+2/3*pi)-u(2)*sin(u(4)+2/3*pi)+u(3)
  abc : Outport
  wires:
  Mux2/1 -> abc/1
  qd2b/1 -> Mux2/2
  qd2a/1 -> Mux2/1
  Mux1/1 -> qd2b/1, qd2c/1, qd2a/1
  theta/1 -> Mux1/2
  dq0/1 -> Mux1/1
  qd2c/1 -> Mux2/3

== system FOC_w_LTID_v2/PMSM motor/dq0 2 abc1 ==
  dq0 : Inport
  theta : Inport  Port=2
  Mux1 : Mux  Inputs=2
  Mux2 : Mux  Inputs=3
  qd2a : Fcn  Expr=u(1)*cos(u(4))-u(2)*sin(u(4))+u(3)
  qd2b : Fcn  Expr=u(1)*cos(u(4)-2/3*pi)-u(2)*sin(u(4)-2/3*pi)+u(3)
  qd2c : Fcn  Expr=u(1)*cos(u(4)+2/3*pi)-u(2)*sin(u(4)+2/3*pi)+u(3)
  abc : Outport
  wires:
  qd2c/1 -> Mux2/3
  dq0/1 -> Mux1/1
  theta/1 -> Mux1/2
  Mux1/1 -> qd2a/1, qd2c/1, qd2b/1
  qd2a/1 -> Mux2/1
  qd2b/1 -> Mux2/2
  Mux2/1 -> abc/1

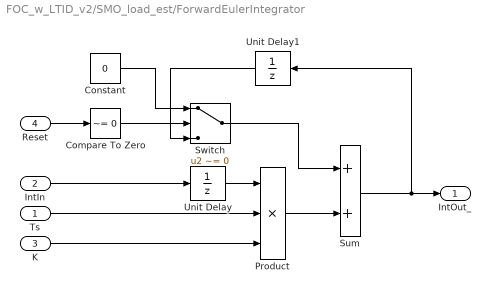
== system FOC_w_LTID_v2/SMO_load_est/ForwardEulerIntegrator ==
  Ts : Inport
  IntIn : Inport  Port=2
  K : Inport  Port=3
  Reset : Inport  Port=4
  Compare To Zero : simulink/Logic and Bit Operations/Compare To Zero  relop=~=  OutDataTypeStr=boolean
  Constant : Constant  Value=0
  Product : Product  Inputs=***
  Sum : Sum
  Switch : Switch  Criteria=u2 ~= 0
  Unit Delay : UnitDelay  SampleTime=-1
  Unit Delay1 : UnitDelay  SampleTime=-1
  IntOut_ : Outport
  wires:
  Sum/1 -> Unit Delay1/1, IntOut_/1
  Reset/1 -> Compare To Zero/1
  Unit Delay/1 -> Product/1
  IntIn/1 -> Unit Delay/1
  K/1 -> Product/3
  Ts/1 -> Product/2
  Constant/1 -> Switch/1
  Compare To Zero/1 -> Switch/2
  Product/1 -> Sum/2
  Switch/1 -> Sum/1
  Unit Delay1/1 -> Switch/3

== system FOC_w_LTID_v2/SMO_load_est/Noise ==
  In1 : Inport
  Constant3 : Constant  Value=noise_ena
  Product2 : Product
  Random Number : RandomNumber  Variance=0.005^2  Seed=21874
  Sum : Sum  Inputs=|++
  Out1 : Outport
  wires:
  In1/1 -> Sum/1
  Sum/1 -> Out1/1
  Product2/1 -> Sum/2
  Random Number/1 -> Product2/1
  Constant3/1 -> Product2/2

== system FOC_w_LTID_v2/SMO_load_est/Noise1 ==
  In1 : Inport
  Constant3 : Constant  Value=noise_ena
  Product2 : Product
  Random Number : RandomNumber  Variance=0.1^2  Seed=86241
  Sum : Sum  Inputs=|++
  Out1 : Outport
  wires:
  In1/1 -> Sum/1
  Sum/1 -> Out1/1
  Product2/1 -> Sum/2
  Random Number/1 -> Product2/1
  Constant3/1 -> Product2/2

== system FOC_w_LTID_v2/SMO_load_est/Subsystem1 ==
  u : Inport
  wn : Inport  Port=2
  Constant : Constant  Value=fs
  MATLAB Function : MATLAB Function  TreatAsAtomicUnit=on
  Memory : Memory  InheritSampleTime=on
  Memory1 : Memory  InheritSampleTime=on
  y : Outport
  wires:
  wn/1 -> MATLAB Function/2(wn)
  Memory1/1 -> MATLAB Function/4(yold)
  Memory/1 -> MATLAB Function/3(uold)
  u/1 -> Memory/1, MATLAB Function/1(u)
  MATLAB Function/1(y) -> Memory1/1, y/1
  Constant/1 -> MATLAB Function/5(fs)

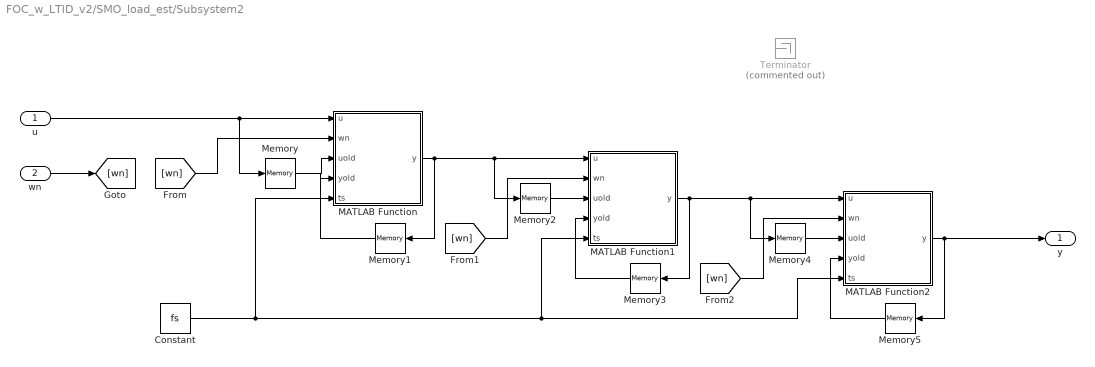
== system FOC_w_LTID_v2/SMO_load_est/Subsystem2 ==
  u : Inport
  wn : Inport  Port=2
  Constant : Constant  Value=fs
  MATLAB Function : MATLAB Function  TreatAsAtomicUnit=on
  MATLAB Function1 : MATLAB Function  TreatAsAtomicUnit=on
  MATLAB Function2 : MATLAB Function  TreatAsAtomicUnit=on
  Memory{,1..5} (6 alike) : Memory  InheritSampleTime=on
  Terminator : Terminator  Commented=on
  y : Outport
  wires:
  Memory1/1 -> MATLAB Function/4(yold)
  Memory/1 -> MATLAB Function/3(uold)
  u/1 -> Memory/1, MATLAB Function/1(u)
  MATLAB Function/1(y) -> Memory2/1, MATLAB Function1/1(u), Memory1/1
  MATLAB Function1/1(y) -> Memory4/1, MATLAB Function2/1(u), Memory3/1
  Memory3/1 -> MATLAB Function1/4(yold)
  Memory2/1 -> MATLAB Function1/3(uold)
  Memory4/1 -> MATLAB Function2/3(uold)
  MATLAB Function2/1(y) -> y/1, Memory5/1
  Memory5/1 -> MATLAB Function2/4(yold)
  wn/1 -> [wn]
  [wn] -> MATLAB Function/2(wn)
  [wn] -> MATLAB Function1/2(wn)
  Constant/1 -> MATLAB Function2/5(ts), MATLAB Function1/5(ts), MATLAB Function/5(ts)
  [wn] -> MATLAB Function2/2(wn)

== system FOC_w_LTID_v2/SMO_load_est/angle to wrapped angle ==
  In_ : Inport
  Atan2 : Trigonometry  Operator=atan2
  Bias1 : Bias  Bias=-pi
  Bias2 : Bias  Bias=-pi
  Bias3 : Bias  Bias=pi
  Cos : Trigonometry  Operator=cos
  Sin : Trigonometry
  Out_ : Outport
  wires:
  Atan2/1 -> Bias3/1
  Bias1/1 -> Sin/1
  Cos/1 -> Atan2/2
  Sin/1 -> Atan2/1
  Bias2/1 -> Cos/1
  Bias3/1 -> Out_/1
  In_/1 -> Bias2/1, Bias1/1

== system FOC_w_LTID_v2/SMO_load_est/saturation ==
  Sigma : Inport
  phi : Inport  Port=2
  Abs : Abs
  Divide : Product  Inputs=*/
  If : If  IfExpression=u1 <= 1
  If Action Subsystem : Subsystem  TreatAsAtomicUnit=on
  If Action Subsystem1 : Subsystem  TreatAsAtomicUnit=on
  Merge : Merge
  Out_ : Outport
  wires:
  Sigma/1 -> If Action Subsystem1/1(In1), Divide/1
  Divide/1 -> If Action Subsystem/1(In1), Abs/1
  phi/1 -> Divide/2
  Abs/1 -> If/1
  If/1 -> If Action Subsystem/Action
  Merge/1 -> Out_/1
  If Action Subsystem/1(Out1) -> Merge/1
  If Action Subsystem1/1(Out1) -> Merge/2
  If/2 -> If Action Subsystem1/Action

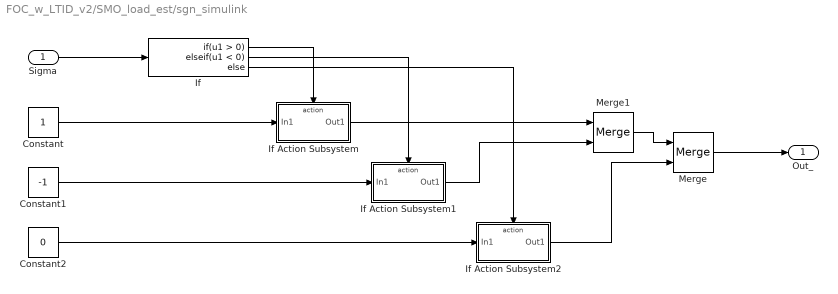
== system FOC_w_LTID_v2/SMO_load_est/sgn_simulink ==
  Sigma : Inport
  Constant : Constant
  Constant1 : Constant  Value=-1
  Constant2 : Constant  Value=0
  If : If  ElseIfExpressions=u1 < 0
  If Action Subsystem : Subsystem  TreatAsAtomicUnit=on
  If Action Subsystem1 : Subsystem  TreatAsAtomicUnit=on
  If Action Subsystem2 : Subsystem  TreatAsAtomicUnit=on
  Merge : Merge
  Merge1 : Merge
  Out_ : Outport
  wires:
  Sigma/1 -> If/1
  Merge/1 -> Out_/1
  Merge1/1 -> Merge/1
  Constant/1 -> If Action Subsystem/1(In1)
  If/1 -> If Action Subsystem/Action
  If Action Subsystem/1(Out1) -> Merge1/1
  Constant1/1 -> If Action Subsystem1/1(In1)
  Constant2/1 -> If Action Subsystem2/1(In1)
  If/2 -> If Action Subsystem1/Action
  If/3 -> If Action Subsystem2/Action
  If Action Subsystem1/1(Out1) -> Merge1/2
  If Action Subsystem2/1(Out1) -> Merge/2

== system FOC_w_LTID_v2/SMO_load_est/sigmoid ==
  Sigma : Inport
  esf : Inport  Port=2
  Abs : Abs
  Divide : Product  Inputs=*/
  Sum : Sum  Inputs=|++
  Out_ : Outport
  wires:
  Abs/1 -> Sum/1
  Sigma/1 -> Divide/1, Abs/1
  Sum/1 -> Divide/2
  esf/1 -> Sum/2
  Divide/1 -> Out_/1

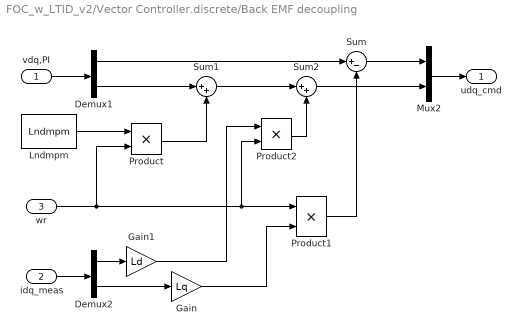
== system FOC_w_LTID_v2/Vector Controller.discrete/Back EMF decoupling ==
  vdq,PI : Inport
  idq_meas : Inport  Port=2
  wr : Inport  Port=3
  Demux1 : Demux  Outputs=2
  Demux2 : Demux  Outputs=2
  Gain : Gain  Gain=Lq
  Gain1 : Gain  Gain=Ld
  Lndmpm : Constant  Value=Lndmpm
  Mux2 : Mux  Inputs=2
  Product : Product  RndMeth=Zero
  Product1 : Product  RndMeth=Zero
  Product2 : Product  RndMeth=Zero
  Sum : Sum  Inputs=|+-
  Sum1 : Sum  Inputs=|++
  Sum2 : Sum  Inputs=|++
  udq_cmd : Outport
  wires:
  Mux2/1 -> udq_cmd/1
  vdq,PI/1 -> Demux1/1
  Demux1/1 -> Sum/1
  Sum/1 -> Mux2/1
  Demux1/2 -> Sum1/1
  idq_meas/1 -> Demux2/1
  wr/1 -> Product/2, Product1/1, Product2/2
  Product1/1 -> Sum/2
  Gain/1 -> Product1/2
  Demux2/2 -> Gain/1
  Lndmpm/1 -> Product/1
  Product/1 -> Sum1/2
  Sum1/1 -> Sum2/1
  Demux2/1 -> Gain1/1
  Gain1/1 -> Product2/1
  Product2/1 -> Sum2/2
  Sum2/1 -> Mux2/2

== system FOC_w_LTID_v2/Vector Controller.discrete/PI controller id ==
  id_err : Inport
  Discrete-Time Integrator : DiscreteIntegrator  SampleTime=-1  ICPrevOutput=DiscIntNeverNeededParam  ICPrevScaledInput=DiscIntNeverNeededParam
  Kp : Gain  Gain=Kp_id
  Sum1 : Sum  Inputs=|++
  ki : Gain  Gain=Ki_id
  vd : Outport
  wires:
  Sum1/1 -> vd/1
  Discrete-Time Integrator/1 -> Sum1/2
  ki/1 -> Discrete-Time Integrator/1
  Kp/1 -> Sum1/1
  id_err/1 -> ki/1, Kp/1

== system FOC_w_LTID_v2/Vector Controller.discrete/PI controller iq ==
  iq_err : Inport
  Discrete-Time Integrator : DiscreteIntegrator  SampleTime=-1  ICPrevOutput=DiscIntNeverNeededParam  ICPrevScaledInput=DiscIntNeverNeededParam
  Kp : Gain  Gain=Kp_iq
  Sum1 : Sum  Inputs=|++
  ki : Gain  Gain=Ki_iq
  vq : Outport
  wires:
  Sum1/1 -> vq/1
  Discrete-Time Integrator/1 -> Sum1/2
  ki/1 -> Discrete-Time Integrator/1
  Kp/1 -> Sum1/1
  iq_err/1 -> ki/1, Kp/1

== system FOC_w_LTID_v2/Vector Controller.discrete/dq 2 afa beta ==
  dq : Inport
  theta : Inport  Port=2
  Mux1 : Mux  Inputs=2
  Mux2 : Mux  Inputs=2
  dq2afa : Fcn  Expr=u(1)*cos(u(3))-u(2)*sin(u(3))
  dq2beta : Fcn  Expr=u(1)*sin(u(3))+u(2)*cos(u(3))
  afa beta : Outport
  wires:
  Mux2/1 -> afa beta/1
  dq2beta/1 -> Mux2/2
  dq2afa/1 -> Mux2/1
  Mux1/1 -> dq2afa/1, dq2beta/1
  theta/1 -> Mux1/2
  dq/1 -> Mux1/1

== system FOC_w_LTID_v2/SMO_load_est/saturation/If Action Subsystem ==
  In1 : Inport
  Action Port : ActionPort  ActionType=then
  Out1 : Outport
  wires:
  In1/1 -> Out1/1

== system FOC_w_LTID_v2/SMO_load_est/saturation/If Action Subsystem1 ==
  In1 : Inport
  Action Port : ActionPort  ActionType=else
  sgn_simulink2 : Subsystem
  Out1 : Outport
  wires:
  In1/1 -> sgn_simulink2/1(Sigma)
  sgn_simulink2/1(Out_) -> Out1/1

== system FOC_w_LTID_v2/SMO_load_est/sgn_simulink/If Action Subsystem ==
  In1 : Inport
  Action Port : ActionPort  ActionType=then
  Out1 : Outport
  wires:
  In1/1 -> Out1/1

== system FOC_w_LTID_v2/SMO_load_est/sgn_simulink/If Action Subsystem1 ==
  In1 : Inport
  Action Port : ActionPort  ActionType=elseif
  Out1 : Outport
  wires:
  In1/1 -> Out1/1

== system FOC_w_LTID_v2/SMO_load_est/sgn_simulink/If Action Subsystem2 ==
  In1 : Inport
  Action Port : ActionPort  ActionType=else
  Out1 : Outport
  wires:
  In1/1 -> Out1/1

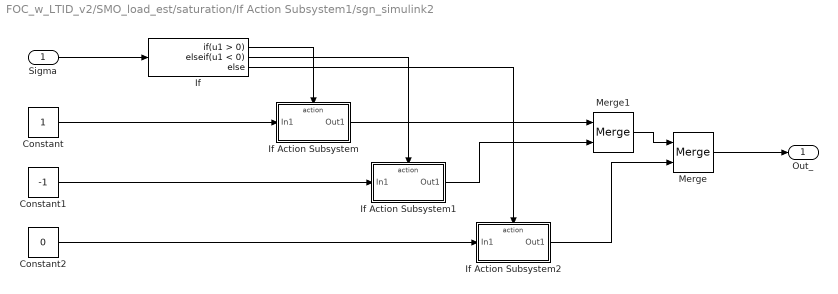
== system FOC_w_LTID_v2/SMO_load_est/saturation/If Action Subsystem1/sgn_simulink2 ==
  Sigma : Inport
  Constant : Constant
  Constant1 : Constant  Value=-1
  Constant2 : Constant  Value=0
  If : If  ElseIfExpressions=u1 < 0
  If Action Subsystem : Subsystem  TreatAsAtomicUnit=on
  If Action Subsystem1 : Subsystem  TreatAsAtomicUnit=on
  If Action Subsystem2 : Subsystem  TreatAsAtomicUnit=on
  Merge : Merge
  Merge1 : Merge
  Out_ : Outport
  wires:
  Sigma/1 -> If/1
  Merge/1 -> Out_/1
  Merge1/1 -> Merge/1
  Constant/1 -> If Action Subsystem/1(In1)
  If/1 -> If Action Subsystem/Action
  If Action Subsystem/1(Out1) -> Merge1/1
  Constant1/1 -> If Action Subsystem1/1(In1)
  Constant2/1 -> If Action Subsystem2/1(In1)
  If/2 -> If Action Subsystem1/Action
  If/3 -> If Action Subsystem2/Action
  If Action Subsystem1/1(Out1) -> Merge1/2
  If Action Subsystem2/1(Out1) -> Merge/2

== system FOC_w_LTID_v2/SMO_load_est/saturation/If Action Subsystem1/sgn_simulink2/If Action Subsystem ==
  In1 : Inport
  Action Port : ActionPort  ActionType=then
  Out1 : Outport
  wires:
  In1/1 -> Out1/1

== system FOC_w_LTID_v2/SMO_load_est/saturation/If Action Subsystem1/sgn_simulink2/If Action Subsystem1 ==
  In1 : Inport
  Action Port : ActionPort  ActionType=elseif
  Out1 : Outport
  wires:
  In1/1 -> Out1/1

== system FOC_w_LTID_v2/SMO_load_est/saturation/If Action Subsystem1/sgn_simulink2/If Action Subsystem2 ==
  In1 : Inport
  Action Port : ActionPort  ActionType=else
  Out1 : Outport
  wires:
  In1/1 -> Out1/1

== matlab function FOC_w_LTID_v2/SMO_load_est/Subsystem2/MATLAB Function ==
  data: u input; y output; wn input; uold input; yold input; ts input
function y = fcn(u,wn, uold, yold, ts)
const = 2*ts;
a1=wn/(wn+const);
a2=(wn-const)/(wn+const);

y=a1*u+a1*uold-a2*yold;

== matlab function FOC_w_LTID_v2/SMO_load_est/Subsystem2/MATLAB Function1 ==
  data: u input; y output; wn input; uold input; yold input; ts input
function y = fcn(u,wn, uold, yold, ts)
const = 2*ts;
a1=wn/(wn+const);
a2=(wn-const)/(wn+const);

y=a1*u+a1*uold-a2*yold;

== matlab function FOC_w_LTID_v2/SMO_load_est/Subsystem2/MATLAB Function2 ==
  data: u input; y output; wn input; uold input; yold input; ts input
function y = fcn(u,wn, uold, yold, ts)
const = 2*ts;
a1=wn/(wn+const);
a2=(wn-const)/(wn+const);

y=a1*u+a1*uold-a2*yold;

== matlab function FOC_w_LTID_v2/SMO_load_est/Subsystem1/MATLAB Function ==
  data: u input; y output; wn input; uold input; yold input; fs input
function y = fcn(u,wn, uold, yold, fs)
a1=wn/(wn+2*fs);
a2=(wn-2*fs)/(wn+2*fs);

y=a1*u+a1*uold-a2*yold;
